simulink model "bench_dcl"  (R2024b)
settings: Solver=daessc  StartTime=0.0  StopTime=10  MaxStep=1e-3  RelTol=1e-3
values from neighbouring files (symbols this model uses):
  PN = evalin('base','PN')    [run_bench_string_heat.m]
libraries: loco_native_lib x7, fl_lib x7, nesl_utility x6
settings Model: Creator=BillBeverley  LastModifiedBy=BillBeverley

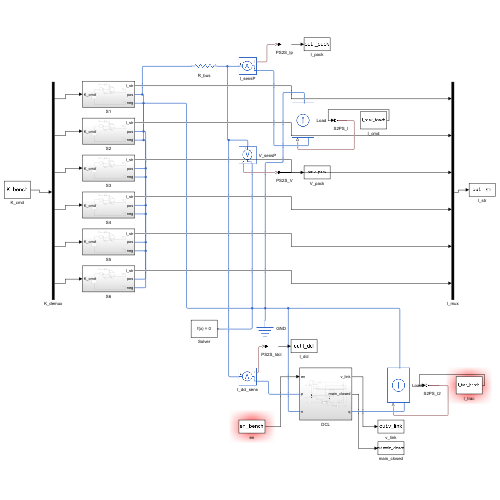
[thumbnail: Simulink's stored preview of the top-level diagram]
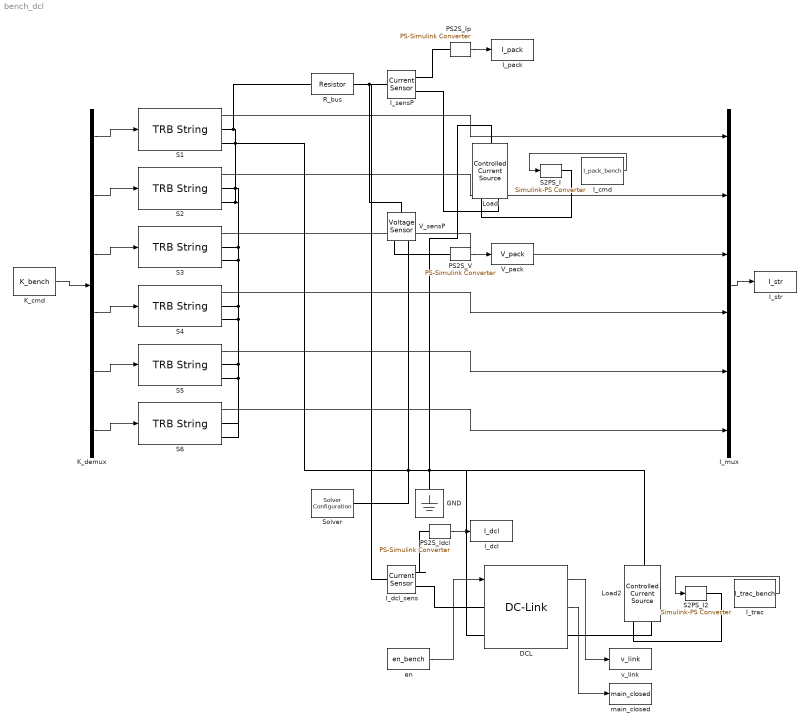
== system bench_dcl ==
  DCL : loco_native_lib/DC-Link  SystemSampleTime=-1  VariantActivationTime=update diagram  AllowFlexibleInterface=on  Latency=0  AutoFrameSizeCalculation=off
  GND : fl_lib/Electrical/Electrical Elements/Electrical Reference
  I_cmd : FromWorkspace  VariableName=I_pack_bench
  I_dcl : ToWorkspace  VariableName=I_dcl  SaveFormat=Timeseries  SampleTime=-1
  I_dcl_sens : fl_lib/Electrical/Electrical Sensors/Current Sensor
  I_mux : Mux  Inputs=6
  I_pack : ToWorkspace  VariableName=I_pack  SaveFormat=Timeseries  SampleTime=-1
  I_sensP : fl_lib/Electrical/Electrical Sensors/Current Sensor
  I_str : ToWorkspace  VariableName=I_str  SaveFormat=Timeseries  SampleTime=-1
  I_trac : FromWorkspace  VariableName=I_trac_bench
  K_cmd : FromWorkspace  VariableName=K_bench
  K_demux : Demux  Outputs=6
  Load : fl_lib/Electrical/Electrical Sources/Controlled Current Source
  Load2 : fl_lib/Electrical/Electrical Sources/Controlled Current Source
  PS2S_Idcl : nesl_utility/PS-Simulink Converter  PhysicalDomain=network_engine_domain  SubClassName=ps_output  LeftPortType=input  RightPortType=output  PseudoPeriodic=off  Frequencies=[]  VectorFormat=inherit  Unit=A  AffineConversion=off
  PS2S_Ip : nesl_utility/PS-Simulink Converter  PhysicalDomain=network_engine_domain  SubClassName=ps_output  LeftPortType=input  RightPortType=output  PseudoPeriodic=off  Frequencies=[]  VectorFormat=inherit  Unit=A  AffineConversion=off
  PS2S_V : nesl_utility/PS-Simulink Converter  PhysicalDomain=network_engine_domain  SubClassName=ps_output  LeftPortType=input  RightPortType=output  PseudoPeriodic=off  Frequencies=[]  VectorFormat=inherit  Unit=V  AffineConversion=off
  R_bus : fl_lib/Electrical/Electrical Elements/Resistor  R=PN.bus.R Ohm  i_specify=off  i_priority=None  i=0 A  i_nominal_specify=off  i_nominal_value=1  i_nominal_unit=A  v_specify=off  v_priority=None  v=0 V  v_nominal_specify=off  v_nominal_value=1  v_nominal_unit=V
  S{1..6} (6 alike) : loco_native_lib/TRB String  SystemSampleTime=-1  VariantActivationTime=update diagram  AllowFlexibleInterface=on  Latency=0  AutoFrameSizeCalculation=off
  S2PS_I : nesl_utility/Simulink-PS Converter  PhysicalDomain=network_engine_domain  SubClassName=ps_input  LeftPortType=input  RightPortType=output  PseudoPeriodic=off  Frequencies=[]  NoiseDistribution=none  NoiseParameters=[]  Unit=A  AffineConversion=off  FilteringAndDerivatives=provide  SimscapeFilterOrder=1  InputFilterTimeConstant=0.001  UdotUserProvided=0
  S2PS_I2 : nesl_utility/Simulink-PS Converter  PhysicalDomain=network_engine_domain  SubClassName=ps_input  LeftPortType=input  RightPortType=output  PseudoPeriodic=off  Frequencies=[]  NoiseDistribution=none  NoiseParameters=[]  Unit=A  AffineConversion=off  FilteringAndDerivatives=provide  SimscapeFilterOrder=1  InputFilterTimeConstant=0.001  UdotUserProvided=0
  Solver : nesl_utility/Solver Configuration  PhysicalDomain=network_engine_domain  SubClassName=solver  LeftPortType=input  RightPortType=generic  Tones=[]  Harmonics=[]  SimulateNoise=off  Profile=off  UseLocalSampling=off  EnableSwitchedLinearOptims=on  FrequencyDomain=off  UseCCode=off  RelTol=0.001  AbsTol=0.001  MinStep=1e-09  ToWorkspace=off  RevertToSquareIcSolve=off  NumHomotopyIterations=100  PhasorMode=off  PhasorModeNumHarmonics=1  ConsistencySolver=NEWTON_XTOL_AFTER_FTOL  IndexReductionMethod=DerivativeReplacement  DoDC=off  ResidualTolerance=1e-09  ConsistencyTolSource=GLOBAL  ConsistencyAbsTol=0.001  ConsistencyRelTol=0.001  ConsistencyTolFactor=0.001  UseLocalSolver=off  LocalSolverChoice=NE_BACKWARD_EULER_ADVANCER  ResolveIndetEquations=on  FunctionEvalNumThread=1  LocalSolverSampleTime=0.001  DoFixedCost=off  MaxNonlinIter=3  MaxModeIter=2  ComputeImpulses=off  ImpulseIterations=2  LinearAlgebra=auto  LinearAlgebraNumThread=0  EquationFormulation=NE_TIME_EF  DelaysMemoryBudget=1024  AutomaticFiltering=on  FilteringTimeConstant=0.001  PartitionStorageMethod=AS_NEEDED  PartitionMemoryBudget=1024  PartitionMethod=ROBUST  MultibodyUseLocalSolver=off  MultibodyLocalSolverChoice=ODE1  MultibodyLocalSolverSampleTime=0.001
  V_pack : ToWorkspace  VariableName=V_pack  SaveFormat=Timeseries  SampleTime=-1
  V_sensP : fl_lib/Electrical/Electrical Sensors/Voltage Sensor
  en : FromWorkspace  VariableName=en_bench
  main_closed : ToWorkspace  VariableName=main_closed  SaveFormat=Timeseries  SampleTime=-1
  v_link : ToWorkspace  VariableName=v_link  SaveFormat=Timeseries  SampleTime=-1
  wires:
  K_cmd/1 -> K_demux/1
  I_mux/1 -> I_str/1
  K_demux/1 -> S1/1
  S1/1 -> I_mux/1
  K_demux/2 -> S2/1
  S2/1 -> I_mux/2
  K_demux/3 -> S3/1
  S3/1 -> I_mux/3
  K_demux/4 -> S4/1
  S4/1 -> I_mux/4
  K_demux/5 -> S5/1
  S5/1 -> I_mux/5
  K_demux/6 -> S6/1
  S6/1 -> I_mux/6
  I_cmd/1 -> S2PS_I/1
  PS2S_Ip/1 -> I_pack/1
  PS2S_V/1 -> V_pack/1
  I_trac/1 -> S2PS_I2/1
  en/1 -> DCL/1
  DCL/1 -> v_link/1
  DCL/2 -> main_closed/1
  PS2S_Idcl/1 -> I_dcl/1
  connections:
  S1/RConn1 -- R_bus/LConn1 -- S2/RConn1 -- S3/RConn1 -- S4/RConn1 -- S5/RConn1 -- S6/RConn1
  R_bus/RConn1 -- I_dcl_sens/LConn1 -- V_sensP/LConn1 -- I_sensP/LConn1
  I_sensP/RConn2 -- Load/RConn2
  S2PS_I/RConn1 -- Load/RConn1
  PS2S_Ip/LConn1 -- I_sensP/RConn1
  PS2S_V/LConn1 -- V_sensP/RConn1
  S1/RConn2 -- Solver/RConn1 -- Load2/LConn1 -- DCL/LConn2 -- GND/LConn1 -- Load/LConn1 -- V_sensP/RConn2 -- S2/RConn2 -- S3/RConn2 -- S4/RConn2 -- S5/RConn2 -- S6/RConn2
  I_dcl_sens/RConn1 -- PS2S_Idcl/LConn1
  I_dcl_sens/RConn2 -- DCL/LConn1
  DCL/RConn1 -- Load2/RConn2
  Load2/RConn1 -- S2PS_I2/RConn1
